simulink model "Q4"  (R2022b)
settings: Solver=ode4  StartTime=0.0  StopTime=50  FixedStep=0.01  RelTol=1e-3
InitFcn:
  | m = 1; % kg
  | k = 1; % N/m
  | b = 0.2;%Ns/m
  | A =  [0, 1;
  |     -k/m, -b/m];
  | B = [0;
  |     1/m];
  | C = [1, 0];
  | D = 0;
undefined symbols (not defined in the file or in its folder): Continuous, Time
libraries: ctrlSharedLib x1, simulink x1
settings Model: Creator=Ali  LastModifiedBy=Ali

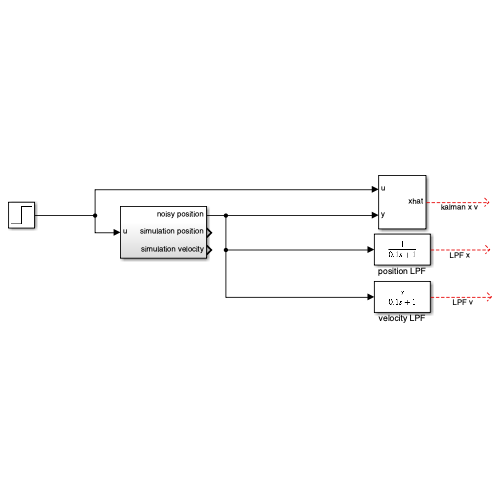
[thumbnail: Simulink's stored preview of the top-level diagram]
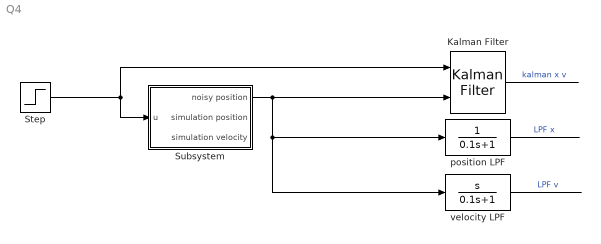
== system Q4 ==
  Kalman Filter : ctrlSharedLib/Kalman Filter  TimeDomain=Continuous-Time  UseCurrentEstimator=on  ModelSource=Individual A, B, C, D matrices  ModelSourceVariable=ss(0.95,1,1,0,1)  A=A  B=B  C=C  D=D  NumberOfStates=1  NumberOfInputs=1  NumberOfOutputs=1  InitialEstimateSource=Dialog  X0=0  P0=10  UseK=off  UseGH=off  NumberOfProcessNoiseInputs=1  G=1  TimeInvariantG=on  H=0  TimeInvariantH=on  Q=0.05  TimeInvariantQ=on  R=1  TimeInvariantR=on  N=0  TimeInvariantN=on  AddInputPort=on  AddEnablePort=off  OutputEstimatedY=off  OutputP=off  Ts=-1
  Step : Step  SampleTime=0
  Subsystem : Subsystem
  position LPF : TransferFcn  Denominator=[0.1 1]
  velocity LPF : TransferFcn  Numerator=[1 0]  Denominator=[0.1 1]
  wires:
  Step/1 -> Kalman Filter/1, Subsystem/1(u)
  Subsystem/1(noisy position) -> velocity LPF/1, position LPF/1, Kalman Filter/2
  position LPF/1 -> ?  "LPF x"
  velocity LPF/1 -> ?  "LPF v"
  Kalman Filter/1 -> ?  "kalman x v"

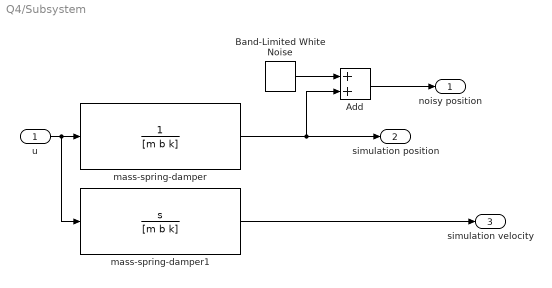
== system Q4/Subsystem ==
  u : Inport
  Add : Sum
  Band-Limited White Noise : simulink/Sources/Band-Limited White Noise  Cov=[0.05]  Ts=0.1  seed=[23341]
  mass-spring-damper : TransferFcn  Denominator=[m b k]
  mass-spring-damper1 : TransferFcn  Numerator=[1 0]  Denominator=[m b k]
  noisy position : Outport
  simulation position : Outport  Port=2
  simulation velocity : Outport  Port=3
  wires:
  mass-spring-damper1/1 -> simulation velocity/1
  u/1 -> mass-spring-damper1/1, mass-spring-damper/1
  mass-spring-damper/1 -> Add/2, simulation position/1
  Band-Limited White Noise/1 -> Add/1
  Add/1 -> noisy position/1
